simulink model "LaoWang_chap9_elec_machinery"  (R2022a)
settings: Solver=VariableStepAuto  StartTime=0.0  StopTime=30  RelTol=1e-3
libraries: Solver_SF x1
settings Model: Creator=HaiChen  LastModifiedBy=HaiChen

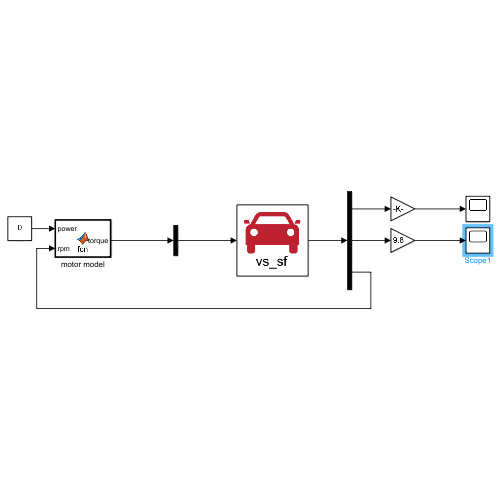
[thumbnail: Simulink's stored preview of the top-level diagram]
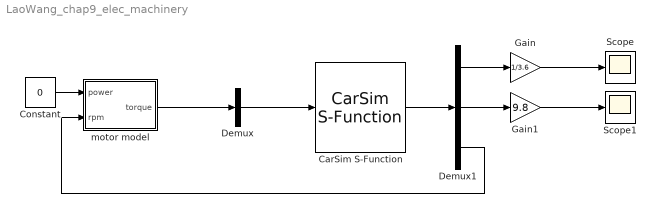
== system LaoWang_chap9_elec_machinery ==
  CarSim S-Function : Solver_SF/CarSim S-Function  Priority=1  SIMFILE=LaoWang_chap9_elec_machinery.sim
  Constant : Constant  Value=0
  Demux : Demux  Outputs=1
  Demux1 : Demux  Outputs=3
  Gain : Gain  Gain=1/3.6
  Gain1 : Gain  Gain=9.8
  Scope : Scope
  Scope1 : Scope
  motor model : MATLAB Function  TreatAsAtomicUnit=on
  wires:
  Demux/1 -> CarSim S-Function/1
  motor model/1(torque) -> Demux/1
  CarSim S-Function/1 -> Demux1/1
  Demux1/1 -> Gain/1
  Demux1/2 -> Gain1/1
  Demux1/3 -> motor model/2(rpm)
  Constant/1 -> motor model/1(power)
  Gain/1 -> Scope/1
  Gain1/1 -> Scope1/1

== matlab function LaoWang_chap9_elec_machinery/motor model ==
  data: power input; torque output; rpm input
function torque = fcn(power,rpm)
    T_max = 380*power;
    if(rpm <= 4523)
        torque = T_max;
    else
        torque = T_max*4523/rpm;
    end
end
